simulink model "FuzzyLogicSimulation"  (R2023a)
settings: Solver=VariableStepAuto  StartTime=0.0  StopTime=10.0  RelTol=1e-3
libraries: simulink x6, spsControlledVoltageSourceLib x1, fuzblock x1, spsPermanentMagnetSynchronousMachineLib x1, spsUniversalBridgeLib x1, spsVoltageMeasurementLib x1, sps_lib x1
settings Model: Creator=Lenovo  LastModifiedBy=hp
settings OptimizationCC: ReuseModelBlockBuffer=off

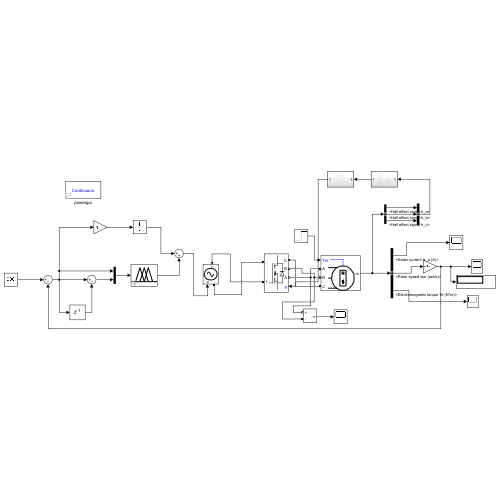
[thumbnail: Simulink's stored preview of the top-level diagram]
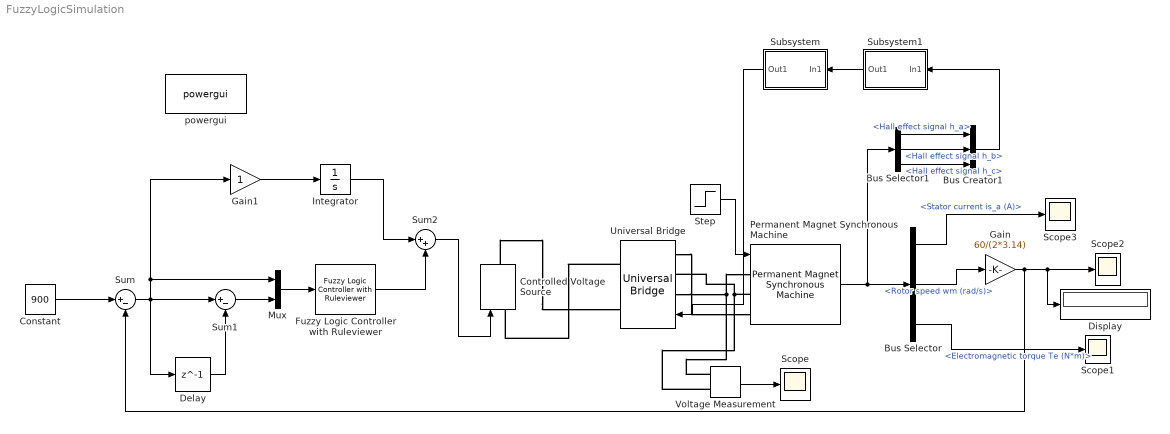
== system FuzzyLogicSimulation ==
  Bus Creator1 : BusCreator  Inputs=3
  Bus Selector : BusSelector  OutputSignals=Stator current is_a (A),Rotor speed wm (rad/s),Electromagnetic torque Te (N*m)
  Bus Selector1 : BusSelector  OutputSignals=Hall effect signal h_a,Hall effect signal h_b,Hall effect signal h_c
  Constant : Constant  Value=900
  Controlled Voltage Source : spsControlledVoltageSourceLib/Controlled Voltage Source  Initialize=on  Source_Type=AC  Amplitude=230  Phase=0  Frequency=50  Measurements=None
  Delay : Delay  DelayLength=1
  Display : Display
  Fuzzy Logic Controller with Ruleviewer : fuzblock/Fuzzy Logic  Controller  with Ruleviewer  fismatrix='RCB'  Ts=2
  Gain : Gain  Gain=60/(2*3.14)
  Gain1 : Gain
  Integrator : Integrator
  Mux : Mux  Inputs=2
  Permanent Magnet Synchronous Machine : spsPermanentMagnetSynchronousMachineLib/Permanent Magnet Synchronous Machine  NbPhases=3  FluxDistribution=Trapezoidal  RotorType=Round  MechanicalLoad=Torque Tm  PresetModel=No  ShowDetailedParameters=on  MeasurementBus=off  Resistance=0.0485  Inductance=8.5e-3  dqInductances=[8.5e-3,8.5e-3]  La=0.000395  MachineConstant=Torque Constant (N.m / A_peak)  Flux=0.1194  VoltageCst=100.0283  TorqueCst=0.9552  Flat=120  Mechanical=[0.0027 0.0004924 4 0]  PolePairs=4  InitialConditions=[0,0, 0,0]  InitialConditions5ph=[0 0 0 0 0 0]  RefAngle=90 degrees behind phase A axis (modified Park)  IterativeDiscreteModel=Trapezoidal non iterative  TsBlock=-1  TsPowergui=0
  Scope{,1..3} (4 alike) : Scope
  Step : Step  SampleTime=0
  Subsystem : Subsystem
  Subsystem1 : Subsystem
  Sum : Sum  Inputs=|+-
  Sum1 : Sum  Inputs=|+-
  Sum2 : Sum  Inputs=|++
  Universal Bridge : spsUniversalBridgeLib/Universal Bridge  Arms=3  SnubberResistance=1e5  SnubberCapacitance=inf  Device=MOSFET / Diodes  Ron=1e-3  Lon=0  ForwardVoltages="[  0  0  ]"  ForwardVoltage=0  GTOparameters=[ 10e-6 , 20e-6 ]  IGBTparameters=[ 1e-6 , 2e-6 ]  Measurements=None  Measurements_2=None  converterType=Rectifier
  Voltage Measurement : spsVoltageMeasurementLib/Voltage Measurement  PhasorSimulation=off  OutputType=Complex  PSBequivalent=0
  powergui : sps_lib/powergui  Priority=1  SimulationMode=Continuous  SampleTime=50e-6  frequency=60  Iterations=50  frequencyindice=50  Pbase=100e6  ErrMax=1e-4  UnitsV=kV  UnitsW=MW  buscounter=0  FunctionMessages=off  echomessages=off  EnableUseOfTLC=off  CurrentSourceSwitches=off  DisableSnubberDevices=off  DisableRonSwitches=off  DisableVfSwitches=off  DisplayEquations=off  AutomaticDiscreteSolvers=off  SolverType=Tustin/Backward Euler (TBE)  Interpol=off  ExternalGateDelay=off  methode=off  Ts=100  x0status=blocks  SPID=on  SwTol=0  HookPort=off  NonlinearTolerance=1e-4  nMaxIteration=100  ContinueOnMaxIteration=off  RestoreLinks=warning  ResistiveCurrentMeasurement=off  Frange=[0:2:500]  Ylog=off  Xlog=on  ShowGrid=off  save=off  variable=ZData  structure=0  ZoomFFT=off  StartTime=0.0  cycles=1  DisplayStyle=1  fundamental=60  FreqAxis=off  MaxFrequency=1000  frequencyindicesteady=1  RmsSteady=1  display=off
  wires:
  Voltage Measurement/1 -> Scope/1
  Permanent Magnet Synchronous Machine/1 -> Bus Selector1/1, Bus Selector/1
  Step/1 -> Permanent Magnet Synchronous Machine/1
  Subsystem1/1(Out1) -> Subsystem/1(In1)
  Subsystem/1(Out1) -> Universal Bridge/1
  Bus Selector/3 -> Scope1/1  "<Electromagnetic torque Te (N*m)>"
  Bus Selector/2 -> Gain/1  "<Rotor speed wm (rad/s)>"
  Gain/1 -> Sum/2, Display/1, Scope2/1
  Bus Selector/1 -> Scope3/1  "<Stator current is_a (A)>"
  Bus Selector1/1 -> Bus Creator1/1  "<Hall effect signal h_a>"
  Bus Selector1/2 -> Bus Creator1/2  "<Hall effect signal h_b>"
  Bus Selector1/3 -> Bus Creator1/3  "<Hall effect signal h_c>"
  Bus Creator1/1 -> Subsystem1/1(In1)
  Sum1/1 -> Mux/2
  Sum/1 -> Delay/1, Mux/1, Gain1/1, Sum1/1
  Constant/1 -> Sum/1
  Delay/1 -> Sum1/2
  Gain1/1 -> Integrator/1
  Integrator/1 -> Sum2/1
  Sum2/1 -> Controlled Voltage Source/1
  Mux/1 -> Fuzzy Logic Controller with Ruleviewer/1
  Fuzzy Logic Controller with Ruleviewer/1 -> Sum2/2
  connections:
  Universal Bridge/LConn1 -- Permanent Magnet Synchronous Machine/LConn1 -- Voltage Measurement/LConn1
  Permanent Magnet Synchronous Machine/LConn2 -- Voltage Measurement/LConn2 -- Universal Bridge/LConn2
  Universal Bridge/LConn3 -- Permanent Magnet Synchronous Machine/LConn3
  Universal Bridge/RConn2 -- Controlled Voltage Source/LConn1
  Controlled Voltage Source/RConn1 -- Universal Bridge/RConn1

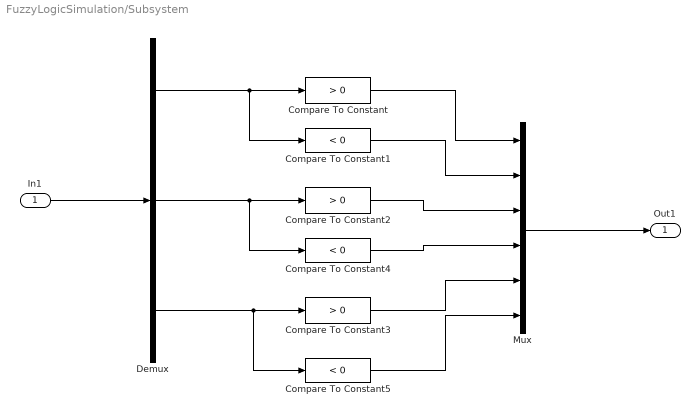
== system FuzzyLogicSimulation/Subsystem ==
  In1 : Inport
  Compare To Constant : simulink/Logic and Bit Operations/Compare To Constant  relop=>  const=0  OutDataTypeStr=boolean
  Compare To Constant1 : simulink/Logic and Bit Operations/Compare To Constant  relop=<  const=0  OutDataTypeStr=boolean
  Compare To Constant2 : simulink/Logic and Bit Operations/Compare To Constant  relop=>  const=0  OutDataTypeStr=boolean
  Compare To Constant3 : simulink/Logic and Bit Operations/Compare To Constant  relop=>  const=0  OutDataTypeStr=boolean
  Compare To Constant4 : simulink/Logic and Bit Operations/Compare To Constant  relop=<  const=0  OutDataTypeStr=boolean
  Compare To Constant5 : simulink/Logic and Bit Operations/Compare To Constant  relop=<  const=0  OutDataTypeStr=boolean
  Demux : Demux  Outputs=3
  Mux : Mux  Inputs=6
  Out1 : Outport
  wires:
  In1/1 -> Demux/1
  Demux/1 -> Compare To Constant1/1, Compare To Constant/1
  Demux/3 -> Compare To Constant5/1, Compare To Constant3/1
  Demux/2 -> Compare To Constant4/1, Compare To Constant2/1
  Compare To Constant/1 -> Mux/1
  Compare To Constant1/1 -> Mux/2
  Compare To Constant2/1 -> Mux/3
  Compare To Constant4/1 -> Mux/4
  Compare To Constant3/1 -> Mux/5
  Compare To Constant5/1 -> Mux/6
  Mux/1 -> Out1/1

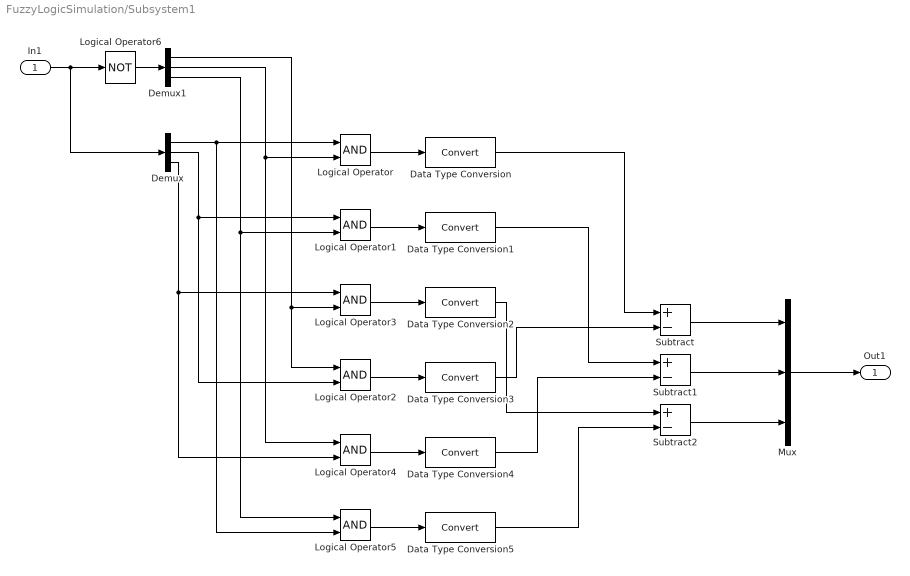
== system FuzzyLogicSimulation/Subsystem1 ==
  In1 : Inport
  Data Type Conversion{,1..5} (6 alike) : DataTypeConversion  SaturateOnIntegerOverflow=off  RndMeth=Floor
  Demux : Demux  Outputs=3
  Demux1 : Demux  Outputs=3
  Logical Operator{,1..5} (6 alike) : Logic  AllPortsSameDT=off  OutDataTypeStr=boolean
  Logical Operator6 : Logic  Operator=NOT  AllPortsSameDT=off  OutDataTypeStr=boolean
  Mux : Mux  Inputs=3
  Subtract : Sum  Inputs=+-
  Subtract1 : Sum  Inputs=+-
  Subtract2 : Sum  Inputs=+-
  Out1 : Outport
  wires:
  In1/1 -> Logical Operator6/1, Demux/1
  Logical Operator6/1 -> Demux1/1
  Logical Operator/1 -> Data Type Conversion/1
  Logical Operator3/1 -> Data Type Conversion2/1
  Logical Operator1/1 -> Data Type Conversion1/1
  Logical Operator2/1 -> Data Type Conversion3/1
  Logical Operator4/1 -> Data Type Conversion4/1
  Logical Operator5/1 -> Data Type Conversion5/1
  Demux/1 -> Logical Operator5/2, Logical Operator/1
  Demux/2 -> Logical Operator1/1, Logical Operator2/2
  Demux/3 -> Logical Operator3/1, Logical Operator4/2
  Demux1/1 -> Logical Operator3/2, Logical Operator2/1
  Demux1/2 -> Logical Operator/2, Logical Operator4/1
  Demux1/3 -> Logical Operator1/2, Logical Operator5/1
  Data Type Conversion5/1 -> Subtract2/2
  Data Type Conversion4/1 -> Subtract1/2
  Data Type Conversion3/1 -> Subtract/2
  Data Type Conversion2/1 -> Subtract2/1
  Data Type Conversion1/1 -> Subtract1/1
  Data Type Conversion/1 -> Subtract/1
  Subtract1/1 -> Mux/2
  Subtract2/1 -> Mux/3
  Subtract/1 -> Mux/1
  Mux/1 -> Out1/1
